simulink model "HILS_ralative"  (R2020a)
settings: Solver=ode4  StartTime=0.0  StopTime=Inf  FixedStep=0.002  RelTol=1e-3
PostLoadFcn:
  | , if any(exist('dsrtsu_mdlpostloadfcn', 'file') == [2, 3, 6]), try dsrtsu_mdlpostloadfcn('Execute', bdroot); catch fprintf('Error in PostLoadFcn (dsrtsu_mdlpostloadfcn) for model "%s":\n %s\n', bdroot, lasterr); end, end,
InitFcn:
  | % mode
  | start_mode = 1;
  | input_mode = 1;
  | HILS_mode = 1;
  | 
  | % input parameter
  | A = 1;
  | Hz = 1;
  | qc = 26500;
  | 
  | % model parameter
  | m1 = 1.5;
  | m2 = 6.4;
  | k1 = 2200;
  | k2 = 405;
  | c1 = 150;
  | c2 = 7;
  | 
  | % convert parameter
  | Gear = 113;
  | enc_pulse = 500;
  | load_to_N = 2;
  | laser_to_mm = 28
  | 
  | % lowpass
  | Cutoff_diff = 20;
  | T_diff = 1/(2*pi*Cutoff_diff);
  | Cutoff_loadcell = 20;
  | T_loadcell = 1/(2*pi*Cutoff_loadcell);
  | Cutoff_laser = 20;
  | T_laser = 1/(2*pi*Cutoff_loadcell);
libraries: rtilib1104 x3, rti1104serlib x2
Description:
  | Standard RTI1104 template.
  | Supported MATLAB version:  R2018a.
settings Model: Tag=RTI1104  DSRTSU_INTERNAL_RTI_VER=520  DSRTSU_INTERNAL_RTI_TYPE=rti1104  RTICANMMDATA=struct('GeneralSetupData',struct('modelroot','C:\Users\VEYRON\Desktop\HILS2020\1DOF_nakagawa\relative','generalsettings',struct('filesettings',struct('destfolder',struct('Name','RTICANMM_FILES','Check',1),'buildfolder',struct('Name','.','Check',1),'AbsDestfolder',struct('Name','C:\Users\VEYRON\Desktop\HILS2020\1DOF_nakagawa\relative\RTICANMM_FILES'),'AbsBuildfolder',struct('Name','C:\Users\VEYRON\Desktop\HILS2020\1DOF_nakagawa\relative'))),'options',struct('addpaths',1,'rmpaths',1,'addtrcexclusion',logical(1),'cannavigator',struct('checkmonitoring',0),'show_usrtrc',0,'use_usrtrc',0),'advanced',struct('options',[1 1 1 1 1 1 1 1 1 1 1 1 1 1 1 1 1 1 1 1 1 1 1 1 1 1 1 1 1 1 1 1 1 1 1 1 1 1 1 1 1 1 1 1 1 1 1 1 1 1 1 1 1 1 1 1 1 1 1 1 1 1 1 1 1 1 1 1 1 1 1 1 1 1 1 1 1 1 1 1 1 1 1 1 1 1 1 1 1 1 1 1 1 1 1 1 1 1 1 1]),'MPSetup',{{}},'modelname','HILS_ralative','block','HILS_ralative'))  DSRTSU_INTERNAL_RTIFLEXRAYCONFIG=110  DSRTSU_INTERNAL_RTIFPGA=110  Creator=VDLAB  LastModifiedBy=Natsu Nakagawa
settings DataIOCC: ReturnWorkspaceOutputs=off
settings OptimizationCC: BlockReduction=off  OptimizeBlockIOStorage=off  BufferReuse=off  GlobalBufferReuse=off  ExpressionFolding=off  LocalBlockOutputs=off  OptimizeDataStoreBuffers=off  BusAssignmentInplaceUpdate=off
settings DebuggingCC: ArithmeticOperatorsInVariantConditions=warning
settings HardwareCC: ProdBitPerPointer=32  ProdBitPerSizeT=32  ProdBitPerPtrDiffT=32  ProdLargestAtomicInteger=Integer  ProdEndianess=BigEndian  ProdWordSize=32  ProdHWDeviceType=Custom Processor->Custom  TargetIntDivRoundTo=Zero  TargetEndianess=BigEndian  TargetHWDeviceType=Custom Processor->Custom
settings SFSimCC: SimUseLocalCustomCode=off  MATLABDynamicMemAlloc=off  CustomCodeUndefinedFunction=UseInterfaceOnly
settings RTWCC: Description=dSPACE DS1104 Hardware Platform  SystemTargetFile=rti1104.tlc  MakeCommand=make_rti  TemplateMakefile=rti1104.tmf  RTWUseLocalCustomCode=off
settings CodeAppCC: StateflowObjectComments=on
settings STFCustomTargetCC: ParMdlRefBuildCompliant=on  SystemTargetFile=rti1104.tlc
settings GRTTargetCC: TargetLangStandard=C89/C90 (ANSI)  CompOptLevelCompliant=off  ConcurrentExecutionCompliant=off  CombineOutputUpdateFcns=off  MatFileLogging=off  CPPClassGenCompliant=off  UseToolchainInfoCompliant=off
settings ConfigComp: CovMetricSettings=dswe

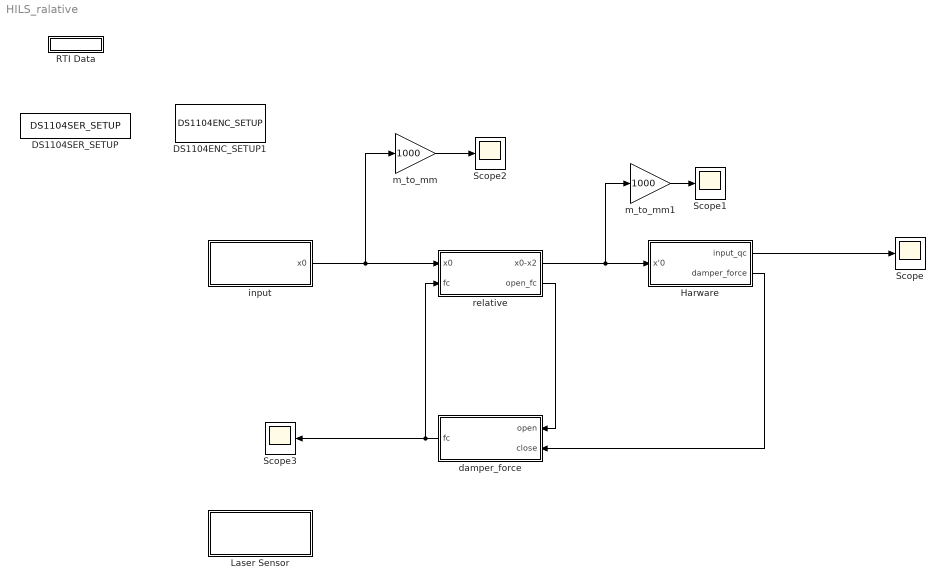
== system HILS_ralative ==
  DS1104ENC_SETUP1 : rtilib1104/DS1104 MASTER PPC/DS1104ENC_SETUP  Reserved1=[]  Reserved2=[]  Reserved3=[]  Reserved4=[]  DialogFcn=gui1104enc_setup  UnitName={'DS1104ENC_SETUP'}  UnitValues={ [] }  DSProperties=struct('RTI',struct('Version',uint32(1),'BlockType',struct('isSLSource',uint8(0),'isSLSink',uint8(0),'isHWSource',uint8(0),'isHWSink',uint8(0),'isSetup',uint8(0),'isInline',uint8(1),'isNonInline',uint8(0),'isInterrupt',uint8(0),'isChannelwise',uint8(0)),'IOBoardType','DS1104MASTER','UnitType','ENC','Identifier','ENCSETUP','DialogType','ML','BlockSet','NONE','SlaveProcessor','NONE'))
      settings: SourceProductName=dSPACE RTI1104  SignalType=[1 1]
  DS1104SER_SETUP : rti1104serlib/DS1104SER_SETUP  Reserved1=[]  Reserved2=[]  Reserved3=[]  Reserved4=[]  DSProperties=struct('RTI',struct('IOBoardType',{{'DS1104','SER'}},'SlaveProcessor','NONE','Version',uint32(2),'BlockType',struct('isSLSource',uint8(0),'isSLSink',uint8(0),'isHWSource',uint8(0),'isHWSink',uint8(0),'isSetup',uint8(1),'isInline',uint8(1),'isNonInline',uint8(0),'isInterrupt',uint8(0),'isChannelwise',uint8(1)),'UnitType','GENSER','Identifier','SETUP','DialogType','ML','BlockSet','NONE'))  RTIBlockInterface=struct('BlockName',struct('Token',{{'DS1104SER_SETUP'}}),'BlockDisplay',{{['Serial Setup'],'center'}},'IconTransparency','off','ParameterTunableNames',{{}},'InitLevel',1,'DialogFcn','guigensersetup','MaskDescription',['To set the global specifications for the UART interface.'])  RTIBlockParameters=struct('ParityMode',{{1,'OFF',[1 5]}},'TransceiverMode',{{1,'OFF',[]}},'QuartzFrequency',{{'16000000','OFF',[1 1]}},'BoardNo',{{1,'ON',[1 1]}},'ChannelNo',{{1,'ON',[1 1]}},'ChannelNumOf',{{1,'OFF',[]}},'BaudRate',{{'115200','OFF',[]}},'DataBitsNumOf',{{4,'OFF',[1 4]}},'StopBitsNumOf',{{1,'OFF',[1 3]}},'ReceiveIntLevelUart',{{4,'OFF',[1 4]}},'AutoflowMode',{{0,'OFF',[]}},'FifoSize',{{'64','OFF',[]}},'ReceiveIntLevelFifo',{{0,'OFF',[]}},'FifoOverrunMode',{{1,'OFF',[]}},'FifoBlockSize',{{'0','OFF',[]}},'TermMode',{{0,'OFF',[]}},'TLCFileName',{{'rtigensersetup','OFF',[]}})  RTISFcnParameters=struct('BoardNo','double','ChannelNo','double','ChannelNumOf','double','BaudRate','double','DataBitsNumOf','double','StopBitsNumOf','double','ParityMode','double','TransceiverMode','double','ReceiveIntLevelUart','double','AutoflowMode','double','FifoSize','double','ReceiveIntLevelFifo','double','FifoBlockSize','double','TermMode','double','QuartzFrequency','double','TLCFileName','char')  RTIBlockParaDefault=struct('ParityMode',1,'TransceiverMode',1,'QuartzFrequency',16000000,'BoardNo',1,'ChannelNo',1,'ChannelNumOf',1,'BaudRate',115200,'DataBitsNumOf',4,'StopBitsNumOf',1,'ReceiveIntLevelUart',4,'AutoflowMode',0,'FifoSize',64,'ReceiveIntLevelFifo',0,'FifoOverrunMode',1,'FifoBlockSize',0,'TermMode',1,'TLCFileName','rtigensersetup')
  Harware : Subsystem
  "Laser Sensor " : Subsystem
  RTI Data : Subsystem  Tag=struct('RTIDataServer',struct('RTIDataServerVs','2','RTIModelDescription','struct(''main'',''HILS_ralative'',''sub'','''',''isMp'',0)'))  LoadFcn="if exist('rtidc'), try,  rtidc('DataHostBlockClbLoad', gcbh); catch, disp(['Warning: ''LoadFcn'' for RTI Data block failed: ' lasterr]); end, end,"  mask(RTI_DATA_HOST){}
      mask help:
      | RTI Data Block.
      | This block is used by RTI to store internal model-dependent data.
      | Please keep this block on the root level of the model. Deleting this block will result in data loss.
      |
      | NEVER DELETE OR COPY THIS BLOCK!
      settings: CopyFcn="if exist('rtidc'), try,  rtidc('DataHostBlockClbCopy', gcbh); catch, disp(['Warning: ''CopyFcn'' for RTI Data block failed: ' lasterr]); end, end,"  DeleteFcn="if exist('rtidc'), try,  rtidc('DataHostBlockClbDelete', gcbh); catch, disp(['Warning: ''DeleteFcn'' for RTI Data block failed: ' lasterr]); end, end,"  ModelCloseFcn="if exist('rtidc'), try,  rtidc('DataHostBlockClbModelClose', gcbh); catch, disp(['Warning: ''ModelCloseFcn'' for RTI Data block failed: ' lasterr]); end, end,"  PreSaveFcn="if exist('rtidc'), try,  rtidc('DataHostBlockClbPreSave', gcbh); catch, disp(['Warning: ''PreSaveFcn'' for RTI Data block failed: ' lasterr]); end, end,"  PostSaveFcn="if exist('rtidc'), try,  rtidc('DataHostBlockClbPostSave', gcbh); catch, disp(['Warning: ''PostSaveFcn'' for RTI Data block failed: ' lasterr]); end, end,"  NameChangeFcn="if exist('rtidc'), try,  rtidc('DataHostBlockClbNameChange', gcbh); catch, disp(['Warning: ''NameChangeFcn'' for RTI Data block failed: ' lasterr]); end, end,"
      mask Help:
      | RTI Data Block.
      | This block is used by RTI to store internal model-dependent data.
      | Please keep this block on the root level of the model. Deleting this block will result in data loss.
      | 
      | NEVER DELETE OR COPY THIS BLOCK!
      mask Display:
      | text(0.5, 0.5, 'RTI Data', 'HorizontalAlignment', 'center');
      | plot([1 0]);
  Scope{,1..3} (4 alike) : Scope
  damper_force : Subsystem
  input : Subsystem
  m_to_mm : Gain  Gain=1000
  m_to_mm1 : Gain  Gain=1000
  relative : Subsystem
  wires:
  input/1(x0) -> m_to_mm/1, relative/1(x0)
  relative/2(open_fc) -> damper_force/1(open)
  damper_force/1(fc) -> Scope3/1, relative/2(fc)
  relative/1(x0-x2) -> m_to_mm1/1, Harware/1(x'0)
  Harware/1(input_qc) -> Scope/1
  Harware/2(damper_force) -> damper_force/2(close)
  m_to_mm/1 -> Scope2/1
  m_to_mm1/1 -> Scope1/1

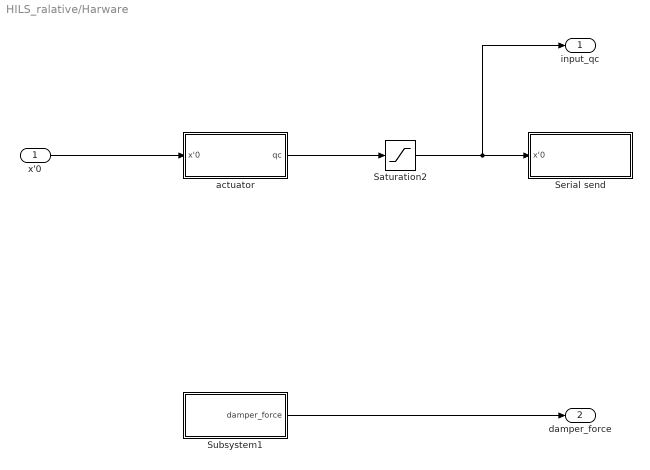
== system HILS_ralative/Harware ==
  x'0 : Inport
  Saturation2 : Saturate  UpperLimit=47000  LowerLimit=0
  Serial send : Subsystem
  Subsystem1 : Subsystem
  actuator : Subsystem
  input_qc : Outport  VectorParamsAs1DForOutWhenUnconnected=off
  damper_force : Outport  Port=2  VectorParamsAs1DForOutWhenUnconnected=off
  wires:
  x'0/1 -> actuator/1(x'0)
  actuator/1(qc) -> Saturation2/1
  Saturation2/1 -> input_qc/1, Serial send/1(x'0)
  Subsystem1/1(damper_force) -> damper_force/1

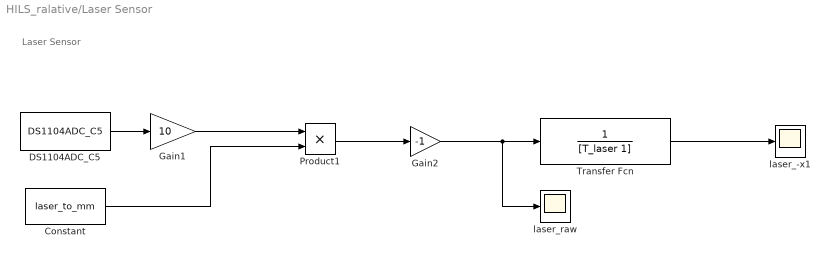
== system HILS_ralative/Laser Sensor  ==
  note: Laser Sensor
  Constant : Constant  Value=laser_to_mm
  DS1104ADC_C5 : rtilib1104/DS1104 MASTER PPC/DS1104ADC_C5  ChannelNo=5  TriggerMode=0  Reserved1=[]  Reserved2=[]  Reserved3=[]  Reserved4=[]  DialogFcn=gui1104adc  UnitName={ 'DS1104ADC_C' }  UnitValues={ 5 }  DSProperties=struct('RTI',struct('Version',uint32(1),'BlockType',struct('isSLSource',uint8(1),'isSLSink',uint8(0),'isHWSource',uint8(1),'isHWSink',uint8(0),'isSetup',uint8(0),'isInline',uint8(1),'isNonInline',uint8(0),'isInterrupt',uint8(0),'isChannelwise',uint8(1)),'IOBoardType','DS1104MASTER','UnitType','ADC','Identifier','ADC','DialogType','ML','BlockSet','NONE','SlaveProcessor','NONE'))
      settings: SourceProductName=dSPACE RTI1104
  Gain1 : Gain  Gain=10
  Gain2 : Gain  Gain=-1
  Product1 : Product
  Transfer Fcn : TransferFcn  Denominator=[T_laser 1]
  laser_-x1 : Scope
  laser_raw : Scope
  wires:
  Gain1/1 -> Product1/1
  Constant/1 -> Product1/2
  DS1104ADC_C5/1 -> Gain1/1
  Product1/1 -> Gain2/1
  Gain2/1 -> laser_raw/1, Transfer Fcn/1
  Transfer Fcn/1 -> laser_-x1/1

== system HILS_ralative/RTI Data ==
  RTI Data Store : Subsystem  Tag="struct('private',struct('version',struct('dsVer',uint32(2),'dsVerCreation',uint32(2),'RTI',struct('ver','7.10','type','RTI1104')),'access',struct('type','Model','isPerm',1,'created',['23-Dec-2020 21:16:23'],'modified',['30-Dec-2020 20:58:09'],'location','')),'public',struct('main',struct('data',[]),'sub',struct('name',{{'HILS_ralative'}},'data',{{struct('TH',struct('thTaskInfo',struct('taskType',{'TIMER','HWINT','TMRINT','SWINT','GLINT'},'tasksNumOf',{1,0,0,0,0},'srcIds',{{'TIMERA'},{},{},{},{}},'taskNames',{{['Timer Task 1']},{},{},{},{}})),'th_tc',struct('dataType','TASK','taskGroupId','','taskGroupList',{{}},'taskSchedulingPolicy','FCFS','taskType','TIMER','blkh',-1,'srcId','TIMERA','srcSgnName',['Timer A interrupt'],'srcCpuName','','taskName',['Timer Task 1  [0.002] s'],'taskNameDisplayExt','','smplTime',0.002,'smplTimeOffs',0,'hasFixedPriority',0,'priority',1,'hasFixedOvc',0,'ovcType',1,'ovcMax',1),'tc_th',struct('dataType','TASK','taskGroupId','','taskGroupList',{{}},'taskSchedulingPolicy','FCFS','taskType','TIMER','blkh',-1,'srcId','TIMERA','srcSgnName',['Timer A interrupt'],'srcCpuName','','taskName',['Timer Task 1  [0.002] s'],'taskNameDisplayExt','','smplTime',0.002,'smplTimeOffs',0,'hasFixedPriority',0,'priority',1,'hasFixedOvc',0,'ovcType',1,'ovcMax',1))}})))"  mask(RTI_DATA_STORE){}
      mask help:
      | RTI Data Store Block. This block is used by RTI to store internal model dependent data. Deleting this block will result in data loss.
      |
      | NEVER DELETE, COPY, OR MODIFY THIS BLOCK!
      mask Help:
      | RTI Data Store Block. This block is used by RTI to store internal model dependent data. Deleting this block will result in data loss.
      | 
      | NEVER DELETE, COPY, OR MODIFY THIS BLOCK!
      mask Display: text(0.5, 0.5, ' ', 'HorizontalAlignment', 'center');

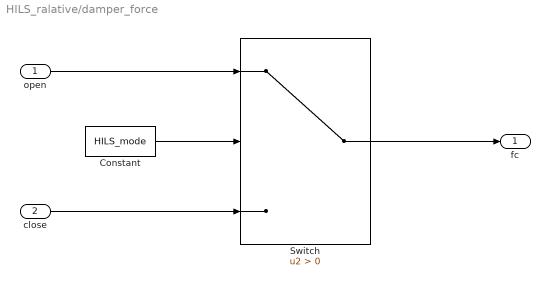
== system HILS_ralative/damper_force ==
  open : Inport
  close : Inport  Port=2
  Constant : Constant  Value=HILS_mode
  Switch : Switch  Criteria=u2 > Threshold
  fc : Outport  VectorParamsAs1DForOutWhenUnconnected=off
  wires:
  open/1 -> Switch/1
  close/1 -> Switch/3
  Constant/1 -> Switch/2
  Switch/1 -> fc/1

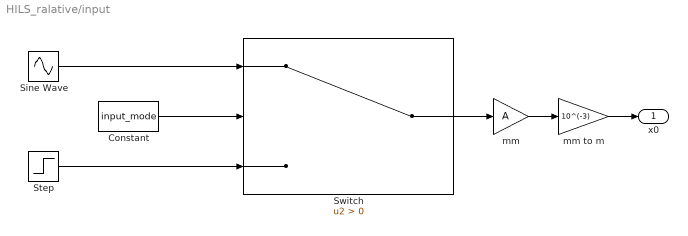
== system HILS_ralative/input ==
  Constant : Constant  Value=input_mode
  Sine Wave : Sin  Frequency=2*pi*Hz  SampleTime=0
  Step : Step  Time=2  SampleTime=0
  Switch : Switch  Criteria=u2 > Threshold
  mm : Gain  Gain=A
  mm to m : Gain  Gain=10^(-3)
  x0 : Outport  VectorParamsAs1DForOutWhenUnconnected=off
  wires:
  Sine Wave/1 -> Switch/1
  Constant/1 -> Switch/2
  Step/1 -> Switch/3
  mm/1 -> mm to m/1
  mm to m/1 -> x0/1
  Switch/1 -> mm/1

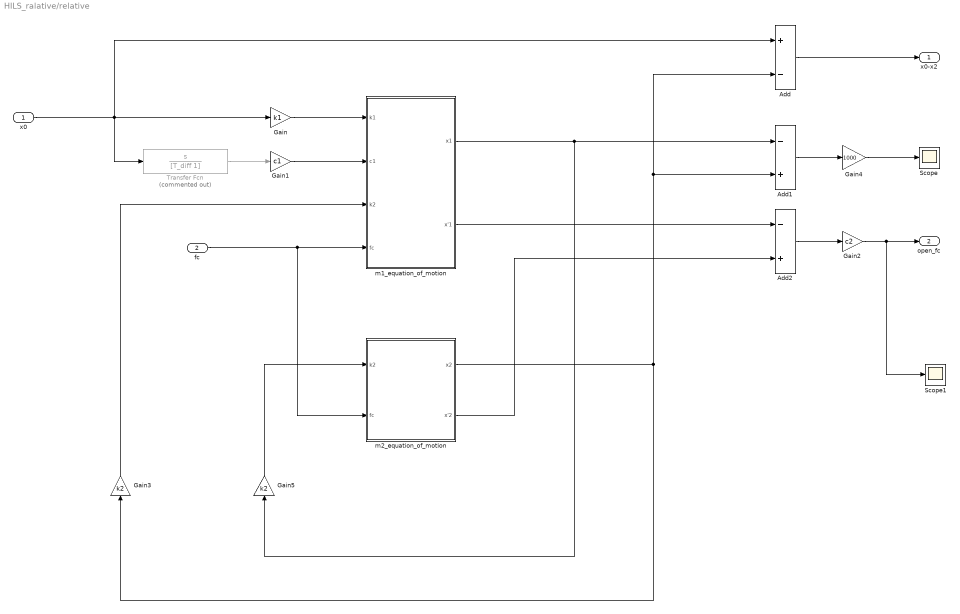
== system HILS_ralative/relative ==
  x0 : Inport
  fc : Inport  Port=2
  Add : Sum  Inputs=+-
  Add1 : Sum  Inputs=-+
  Add2 : Sum  Inputs=-+
  Gain : Gain  Gain=k1
  Gain1 : Gain  Gain=c1
  Gain2 : Gain  Gain=c2
  Gain3 : Gain  Gain=k2
  Gain4 : Gain  Gain=1000
  Gain5 : Gain  Gain=k2
  Scope : Scope
  Scope1 : Scope
  Transfer Fcn : TransferFcn  Commented=on  Numerator=[1 0]  Denominator=[T_diff 1]
  m1_equation_of_motion : Subsystem
  m2_equation_of_motion : Subsystem
  x0-x2 : Outport  VectorParamsAs1DForOutWhenUnconnected=off
  open_fc : Outport  Port=2  VectorParamsAs1DForOutWhenUnconnected=off
  wires:
  x0/1 -> Gain/1, Add/1, Transfer Fcn/1
  Gain/1 -> m1_equation_of_motion/1(k1)
  Transfer Fcn/1 -> Gain1/1
  Gain1/1 -> m1_equation_of_motion/2(c1)
  m2_equation_of_motion/2(x'2) -> Add2/2
  m2_equation_of_motion/1(x2) -> Add1/2, Add/2, Gain3/1
  Gain3/1 -> m1_equation_of_motion/3(k2)
  m1_equation_of_motion/2(x'1) -> Add2/1
  Gain5/1 -> m2_equation_of_motion/1(k2)
  m1_equation_of_motion/1(x1) -> Add1/1, Gain5/1
  Add/1 -> x0-x2/1
  Add1/1 -> Gain4/1
  fc/1 -> m2_equation_of_motion/2(fc), m1_equation_of_motion/4(fc)
  Add2/1 -> Gain2/1
  Gain2/1 -> Scope1/1, open_fc/1
  Gain4/1 -> Scope/1

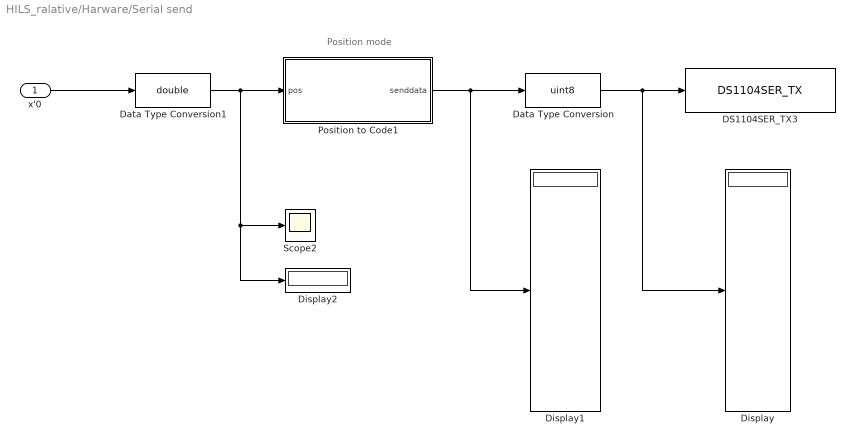
== system HILS_ralative/Harware/Serial send ==
  note: Position mode
  x'0 : Inport
  DS1104SER_TX3 : rti1104serlib/DS1104SER_TX  Reserved1=[]  Reserved2=[]  Reserved3=[]  Reserved4=[]  DSProperties=struct('RTI',struct('IOBoardType',{{'DS1104','SER'}},'SlaveProcessor','NONE','Version',uint32(1),'BlockType',struct('isSLSource',uint8(1),'isSLSink',uint8(1),'isHWSource',uint8(1),'isHWSink',uint8(0),'isSetup',uint8(0),'isInline',uint8(1),'isNonInline',uint8(0),'isInterrupt',uint8(0),'isChannelwise',uint8(1)),'UnitType','GENSER','Identifier','TRANSMIT','DialogType','ML','BlockSet','NONE'))  RTIBlockInterface=struct('BlockName',struct('Token',{{'DS1104SER_TX'}}),'InputPortsWidth',int32([14 1]),'InputPortsActive',[1 0],'InputPortsDataType',{{'SS_UINT8','SS_UINT32'}},'InputPortsName',{{'TXBytes','NumBytes'}},'OutputPortsWidth',int32([1 1]),'OutputPortsActive',[0 0],'OutputPortsDataType',{{'SS_UINT32','SS_INT32'}},'OutputPortsName',{{'NumTXBytes','Status'}},'BlockDisplay',{{['Serial Transmit'],'center'}},'IconTransparency','on','ParameterTunableNames',{{}},'InitLevel',2,'DialogFcn','guigensertransmit','MaskDescription',['To write data to the UART SW FIFO.'])  RTIBlockParameters=struct('BoardNo',{{1,'ON',[1 1]}},'ChannelNo',{{1,'ON',[1 1]}},'ChannelNumOf',{{1,'OFF',[]}},'TransmitFifoOverrunMode',{{1,'OFF',[]}},'ParamTunableMode',{{2,'OFF',[]}},'BytesRefNumOfT',{{'1','OFF',[1 inf]}},'BytesRefNumOfNT',{{'14','OFF',[1 inf]}},'BytesRefNumOfMax',{{'1','OFF',[1 inf]}},'BytesRefNumOfMode',{{0,'OFF',[]}},'BytesActNumOfMode',{{0,'OFF',[]}},'TransmissionStatusMode',{{0,'OFF',[]}},'FifoSizeDefault',{{64,'OFF',[]}},'TLCFileName',{{'rtigensertransmit','OFF',[]}})  RTISFcnParameters=struct('BoardNo','double','ChannelNo','double','ChannelNumOf','double','TransmitFifoOverrunMode','double','ParamTunableMode','double','BytesRefNumOfT','double','BytesRefNumOfNT','double','BytesRefNumOfMax','double','BytesRefNumOfMode','double','BytesActNumOfMode','double','TransmissionStatusMode','double','TLCFileName','char')  RTIBlockParaDefault=struct('BoardNo',1,'ChannelNo',1,'ChannelNumOf',1,'TransmitFifoOverrunMode',1,'ParamTunableMode',1,'BytesRefNumOfT',1,'BytesRefNumOfNT',1,'BytesRefNumOfMax',1,'BytesRefNumOfMode',0,'BytesActNumOfMode',1,'TransmissionStatusMode',1,'FifoSizeDefault',64,'TLCFileName','rtigensertransmit')
  Data Type Conversion : DataTypeConversion  OutDataTypeStr=uint8
  Data Type Conversion1 : DataTypeConversion  OutDataTypeStr=double  RndMeth=Ceiling
  Display : Display
  Display1 : Display
  Display2 : Display
  Position to Code1 : MATLAB Function  TreatAsAtomicUnit=on
  Scope2 : Scope
  wires:
  Data Type Conversion1/1 -> Position to Code1/1(pos), Scope2/1, Display2/1
  Position to Code1/1(senddata) -> Data Type Conversion/1, Display1/1
  Data Type Conversion/1 -> DS1104SER_TX3/1, Display/1
  x'0/1 -> Data Type Conversion1/1

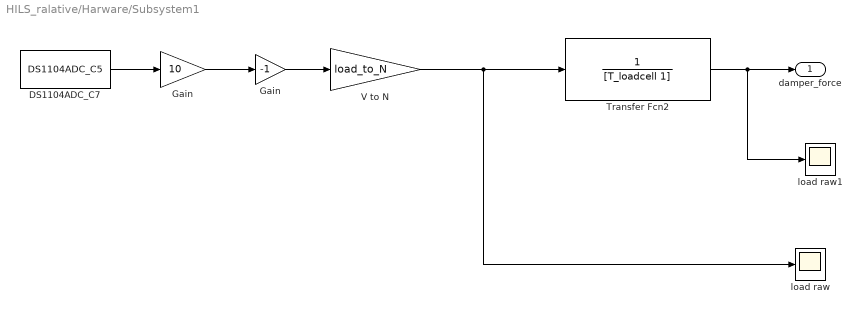
== system HILS_ralative/Harware/Subsystem1 ==
  DS1104ADC_C7 : rtilib1104/DS1104 MASTER PPC/DS1104ADC_C5  ChannelNo=7  TriggerMode=0  Reserved1=[]  Reserved2=[]  Reserved3=[]  Reserved4=[]  DialogFcn=gui1104adc  UnitName={ 'DS1104ADC_C' }  UnitValues={ 7 }  DSProperties=struct('RTI',struct('Version',uint32(1),'BlockType',struct('isSLSource',uint8(1),'isSLSink',uint8(0),'isHWSource',uint8(1),'isHWSink',uint8(0),'isSetup',uint8(0),'isInline',uint8(1),'isNonInline',uint8(0),'isInterrupt',uint8(0),'isChannelwise',uint8(1)),'IOBoardType','DS1104MASTER','UnitType','ADC','Identifier','ADC','DialogType','ML','BlockSet','NONE','SlaveProcessor','NONE'))
      settings: SourceProductName=dSPACE RTI1104
  Gain : Gain  Gain=-1
  "Gain " : Gain  Gain=10
  Transfer Fcn2 : TransferFcn  Denominator=[T_loadcell 1]
  V to N : Gain  Gain=load_to_N
  load raw : Scope
  load raw1 : Scope
  damper_force : Outport  VectorParamsAs1DForOutWhenUnconnected=off
  wires:
  Gain/1 -> V to N/1
  "Gain "/1 -> Gain/1
  DS1104ADC_C7/1 -> "Gain "/1
  V to N/1 -> load raw/1, Transfer Fcn2/1
  Transfer Fcn2/1 -> load raw1/1, damper_force/1

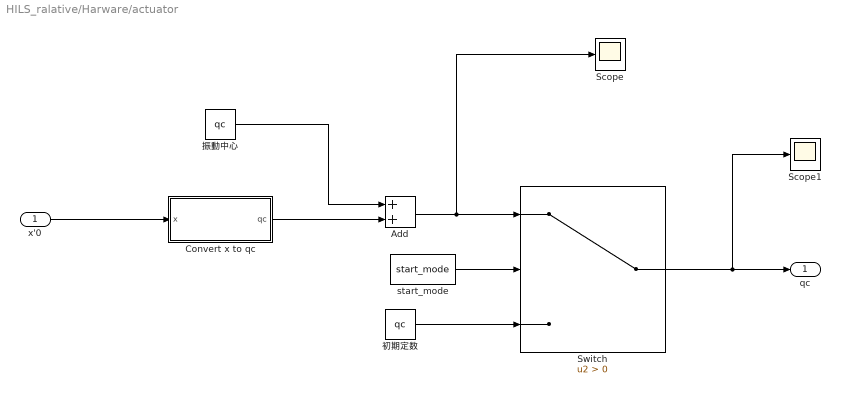
== system HILS_ralative/Harware/actuator ==
  x'0 : Inport
  Add : Sum
  Convert x to qc : Subsystem
  Scope : Scope
  Scope1 : Scope
  Switch : Switch  Criteria=u2 > Threshold
  start_mode : Constant  Value=start_mode
  初期定数 : Constant  Value=qc
  振動中心 : Constant  Value=qc
  qc : Outport  VectorParamsAs1DForOutWhenUnconnected=off
  wires:
  x'0/1 -> Convert x to qc/1(x)
  初期定数/1 -> Switch/3
  Switch/1 -> Scope1/1, qc/1
  start_mode/1 -> Switch/2
  Convert x to qc/1(qc) -> Add/2
  Add/1 -> Scope/1, Switch/1
  振動中心/1 -> Add/1

== system HILS_ralative/RTI Data/RTI Data Store ==
  RTI Data Store : Subsystem  mask(RTI_DATA_STORE){}
      mask help:
      | RTI Data Store Block. This block is used by RTI to store internal model dependent data. Deleting this block will result in data loss.
      |
      | NEVER DELETE, COPY, OR MODIFY THIS BLOCK!
      mask Help:
      | RTI Data Store Block. This block is used by RTI to store internal model dependent data. Deleting this block will result in data loss.
      | 
      | NEVER DELETE, COPY, OR MODIFY THIS BLOCK!
      mask Display: text(0.5, 0.5, ' ', 'HorizontalAlignment', 'center');

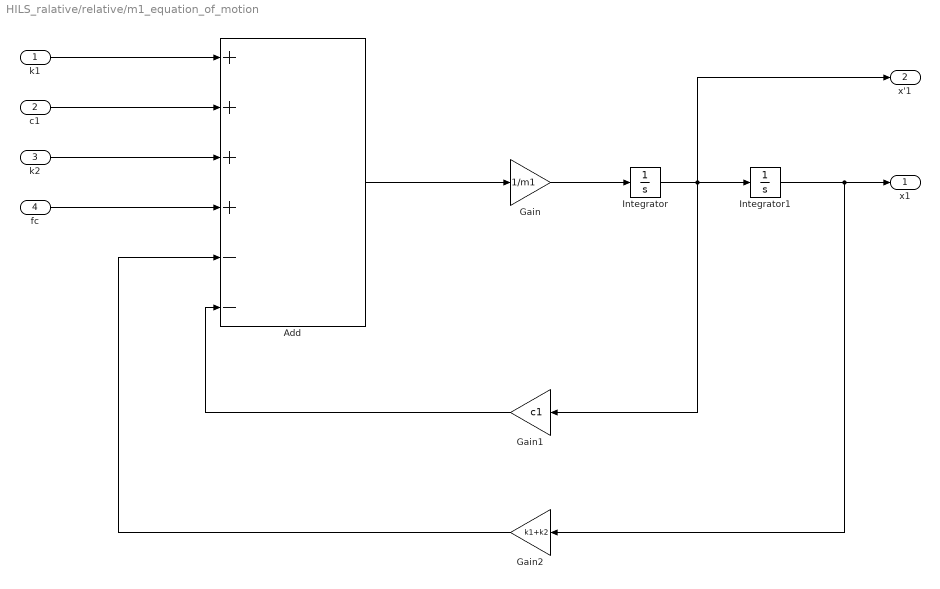
== system HILS_ralative/relative/m1_equation_of_motion ==
  k1 : Inport
  c1 : Inport  Port=2
  k2 : Inport  Port=3
  fc : Inport  Port=4
  Add : Sum  Inputs=++++--
  Gain : Gain  Gain=1/m1
  Gain1 : Gain  Gain=c1
  Gain2 : Gain  Gain=k1+k2
  Integrator : Integrator
  Integrator1 : Integrator
  x1 : Outport  VectorParamsAs1DForOutWhenUnconnected=off
  x'1 : Outport  Port=2  VectorParamsAs1DForOutWhenUnconnected=off
  wires:
  k1/1 -> Add/1
  c1/1 -> Add/2
  k2/1 -> Add/3
  fc/1 -> Add/4
  Add/1 -> Gain/1
  Gain/1 -> Integrator/1
  Integrator/1 -> Integrator1/1, x'1/1, Gain1/1
  Integrator1/1 -> Gain2/1, x1/1
  Gain1/1 -> Add/6
  Gain2/1 -> Add/5

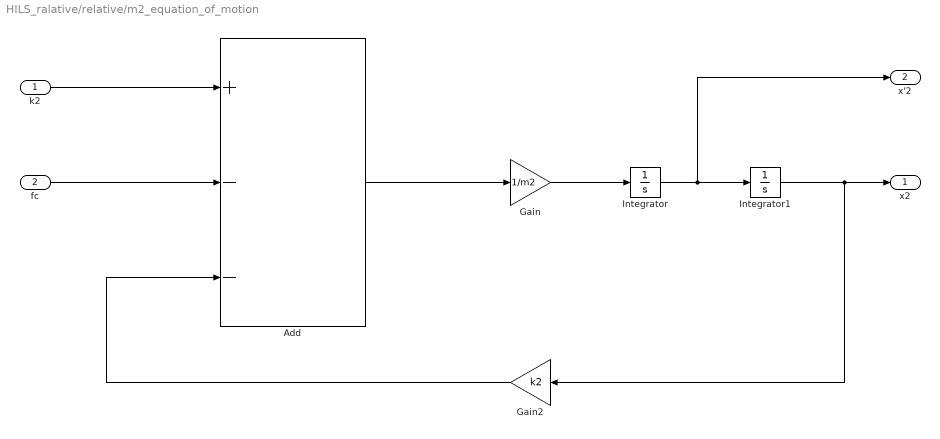
== system HILS_ralative/relative/m2_equation_of_motion ==
  k2 : Inport
  fc : Inport  Port=2
  Add : Sum  Inputs=+--
  Gain : Gain  Gain=1/m2
  Gain2 : Gain  Gain=k2
  Integrator : Integrator
  Integrator1 : Integrator
  x2 : Outport  VectorParamsAs1DForOutWhenUnconnected=off
  x'2 : Outport  Port=2  VectorParamsAs1DForOutWhenUnconnected=off
  wires:
  k2/1 -> Add/1
  fc/1 -> Add/2
  Add/1 -> Gain/1
  Gain/1 -> Integrator/1
  Integrator/1 -> Integrator1/1, x'2/1
  Integrator1/1 -> Gain2/1, x2/1
  Gain2/1 -> Add/3

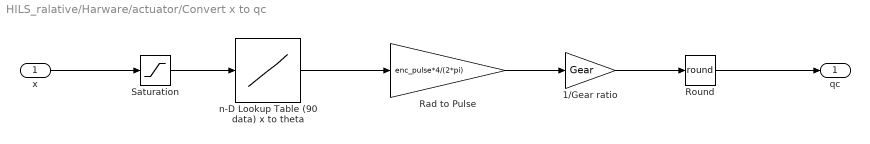
== system HILS_ralative/Harware/actuator/Convert x to qc ==
  x : Inport
  1/Gear ratio : Gain  Gain=Gear
  Rad to Pulse : Gain  Gain=enc_pulse*4/(2*pi)
  Round : Rounding  Operator=round
  Saturation : Saturate  UpperLimit=0.38  LowerLimit=-0.25
  n-D Lookup Table (90 data) x to theta : Lookup_n-D  NumberOfTableDimensions=1  BreakpointsForDimension1=|  BreakpointsForDimension3=[5, 7]  Table=|  InterpMethod=Cubic spline  ExtrapMethod=Cubic spline  InternalRulePriority=Speed  RndMeth=Simplest  InputSameDT=on
      BreakpointsForDimension1=|
      | [-0.0255748
      | -0.025224748
      | -0.024865444
      | -0.024496806
      | -0.024118754
      | -0.023731207
      | -0.023334088
      | -0.022927321
      | -0.022510829
      | -0.022084541
      | -0.021648387
      | -0.021202299
      | -0.020746214
      | -0.02028007
      | -0.01980381
      | -0.019317383
      | -0.018820738
      | -0.018313834
      | -0.01779663
      | -0.017269095
      | -0.016731201
      | -0.016182927
      | -0.015624258
      | -0.015055189
      | -0.014475717
      | -0.013885852
      | -0.013285608
      | -0.012675011
      | -0.012054093
      | -0.011422895
      | -0.010781471
      | -0.01012988
      | -0.009468194
      | -0.008796496
      | -0.008114876
      | -0.007423439
      | -0.006722299
      | -0.006011582
      | -0.005291424
      | -0.004561974
      | -0.003823394
      | -0.003075856
      | -0.002319545
      | -0.001554657
      | -0.000781402
      | 0
      | 0.000789315
      | 0.001586298
      | 0.002390691
      | 0.003202226
      | 0.004020623
      | 0.004845587
      | 0.005676817
      | 0.006513997
      | 0.007356803
      | 0.008204897
      | 0.009057933
      | 0.009915556
      | 0.010777401
      | 0.011643091
      | 0.012512243
      | 0.013384467
      | 0.014259361
      | 0.015136519
      | 0.016015526
      | 0.016895961
      | 0.017777398
      | 0.018659405
      | 0.019541543
      | 0.020423371
      | 0.021304443
      | 0.022184308
      | 0.023062515
      | 0.023938607
      | 0.024812127
      | 0.025682617
      | 0.026549617
      | 0.027412664
      | 0.0282713
      | 0.029125062
      | 0.029973492
      | 0.030816132
      | 0.031652523
      | 0.032482212
      | 0.033304747
      | 0.034119678
      | 0.034926559
      | 0.035724949
      | 0.036514409
      | 0.037294505
      | 0.03806481
      | ]
      Table=|
      | [-0.785398163
      | -0.767944871
      | -0.750491578
      | -0.733038286
      | -0.715584993
      | -0.698131701
      | -0.680678408
      | -0.663225116
      | -0.645771823
      | -0.628318531
      | -0.610865238
      | -0.593411946
      | -0.575958653
      | -0.558505361
      | -0.541052068
      | -0.523598776
      | -0.506145483
      | -0.488692191
      | -0.471238898
      | -0.453785606
      | -0.436332313
      | -0.41887902
      | -0.401425728
      | -0.383972435
      | -0.366519143
      | -0.34906585
      | -0.331612558
      | -0.314159265
      | -0.296705973
      | -0.27925268
      | -0.261799388
      | -0.244346095
      | -0.226892803
      | -0.20943951
      | -0.191986218
      | -0.174532925
      | -0.157079633
      | -0.13962634
      | -0.122173048
      | -0.104719755
      | -0.087266463
      | -0.06981317
      | -0.052359878
      | -0.034906585
      | -0.017453293
      | 0
      | 0.017453293
      | 0.034906585
      | 0.052359878
      | 0.06981317
      | 0.087266463
      | 0.104719755
      | 0.122173048
      | 0.13962634
      | 0.157079633
      | 0.174532925
      | 0.191986218
      | 0.20943951
      | 0.226892803
      | 0.244346095
      | 0.261799388
      | 0.27925268
      | 0.296705973
      | 0.314159265
      | 0.331612558
      | 0.34906585
      | 0.366519143
      | 0.383972435
      | 0.401425728
      | 0.41887902
      | 0.436332313
      | 0.453785606
      | 0.471238898
      | 0.488692191
      | 0.506145483
      | 0.523598776
      | 0.541052068
      | 0.558505361
      | 0.575958653
      | 0.593411946
      | 0.610865238
      | 0.628318531
      | 0.645771823
      | 0.663225116
      | 0.680678408
      | 0.698131701
      | 0.715584993
      | 0.733038286
      | 0.750491578
      | 0.767944871
      | 0.785398163
      | ]
  qc : Outport  VectorParamsAs1DForOutWhenUnconnected=off
  wires:
  x/1 -> Saturation/1
  Saturation/1 -> n-D Lookup Table (90 data) x to theta/1
  n-D Lookup Table (90 data) x to theta/1 -> Rad to Pulse/1
  Rad to Pulse/1 -> 1/Gear ratio/1
  1/Gear ratio/1 -> Round/1
  Round/1 -> qc/1

== system HILS_ralative/RTI Data/RTI Data Store/RTI Data Store ==
  RTI Data Store : Subsystem  mask(RTI_DATA_STORE){}
      mask help:
      | RTI Data Store Block. This block is used by RTI to store internal model dependent data. Deleting this block will result in data loss.
      |
      | NEVER DELETE, COPY, OR MODIFY THIS BLOCK!
      mask Help:
      | RTI Data Store Block. This block is used by RTI to store internal model dependent data. Deleting this block will result in data loss.
      | 
      | NEVER DELETE, COPY, OR MODIFY THIS BLOCK!
      mask Display: text(0.5, 0.5, ' ', 'HorizontalAlignment', 'center');

== system HILS_ralative/RTI Data/RTI Data Store/RTI Data Store/RTI Data Store ==
  RTI Data Store : Subsystem  mask(RTI_DATA_STORE){}
      mask help:
      | RTI Data Store Block. This block is used by RTI to store internal model dependent data. Deleting this block will result in data loss.
      |
      | NEVER DELETE, COPY, OR MODIFY THIS BLOCK!
      mask Help:
      | RTI Data Store Block. This block is used by RTI to store internal model dependent data. Deleting this block will result in data loss.
      | 
      | NEVER DELETE, COPY, OR MODIFY THIS BLOCK!
      mask Display: text(0.5, 0.5, ' ', 'HorizontalAlignment', 'center');

== system HILS_ralative/RTI Data/RTI Data Store/RTI Data Store/RTI Data Store/RTI Data Store ==

== matlab function HILS_ralative/Harware/Serial send/Position to Code1 ==
  data: pos input; senddata output
% script_sendTargetPosition
% MATLAB EPOS LibraryのsendTargetPosition()から書き換え

% function [] = sendTargetPosition( obj, pos )

function senddata = func_sendTargetPosition(pos)
% pos = 20480;

%Sets the TargetPosition for Profile Position mode
%pos must be an integer.
pos_hex = '';

if pos >= 0
    pos_hex = dec2hex(pos, 8);
else
    pos_hex = dec2hex(2^32+pos, 8);
end

%% Build write object request frame EPOS Node 1
%opCode(write): 0x11
%Len-1: 3
%object index(Target Position): 0x2062
%subindex and nodeID: 0x0100
%BYTE Data[4]: pos_hex(1:4), pos_hex(5:8)


%opCode = uint16(myhex2dec('11'));
opCode = uint16(17);
Len_1 = uint16(3);
%DATA = uint16([myhex2dec('62') myhex2dec('20') myhex2dec('00') myhex2dec('01') myhex2dec(pos_hex(7:8))
%   myhex2dec(pos_hex(5:6)) 
%   myhex2dec(pos_hex(3:4)) myhex2dec(pos_hex(1:2)) ]);
DATA = uint16([98 32 0 1 myhex2dec(pos_hex(7:8)) myhex2dec(pos_hex(5:6)) myhex2dec(pos_hex(3:4)) myhex2dec(pos_hex(1:2)) ]);
%DATAforCRC = uint16([myhex2dec('1103') myhex2dec('2062') myhex2dec('0100') myhex2dec(pos_hex(5:8)) 
%   myhex2dec(pos_hex(1:4)) myhex2dec('0000')]);
DATAforCRC = uint16([4355 8290 256 myhex2dec(pos_hex(5:8)) myhex2dec(pos_hex(1:4)) 0]);
numberofWordsCRC = 6;
crc_hex = dec2hex(CRCcalc(DATAforCRC, numberofWordsCRC),4);
CRC = uint16([myhex2dec(crc_hex(3:4)) myhex2dec(crc_hex(1:2))]);

% senddata=[opCode Len_1 DATA CRC char('O')];
senddata=[opCode Len_1 DATA CRC 79 10]';

end


function d = myhex2dec(h)
%HEX2DEC Convert hexadecimal string to decimal integer.
%   this is the hex2dec function from Matlab with some checking disabled
%   for faster performance

if iscellstr(h), h = char(h); end
if isempty(h), d = []; return, end

% Work in upper case. - disabled since upper case anyways
%h = upper(h);

[m,n]=size(h);

% Right justify strings and form 2-D character array.
if ~isempty(find((h==' ' | h==0),1))
  h = strjust(h);

  % Replace any leading blanks and nulls by 0.
  h(cumsum(h ~= ' ' & h ~= 0,2) == 0) = '0';
else
  h = reshape(h,m,n);
end

% Check for out of range values - disabled
% if any(any(~((h>='0' & h<='9') | (h>='A'&h<='F'))))
%    error(message('MATLAB:hex2dec:IllegalHexadecimal'));
% end

sixteen = 16;
p = fliplr(cumprod([1 sixteen(ones(1,n-1))]));
p = p(ones(m,1),:);

d = h <= 64; % Numbers
h(d) = h(d) - 48;

d =  h > 64; % Letters
h(d) = h(d) - 55;

d = sum(h.*p,2);


end

function [ CRC ] = CRCcalc(DataArray, CRCnumberOfWords)
%Calculates the 16 bit CRC checksum according to communication guide for
%EPOS2
%Arguments are the DataArray that is being sent (opCode to Data) and the
%number of words

CRC = uint16(0);
for i=1:CRCnumberOfWords
    
    %shifter = uint16(myhex2dec('8000'));
    shifter = uint16(32768);
    c = DataArray(i);
    
    while(shifter)
        %carry = bitand(CRC, uint16(myhex2dec('8000')), 'uint16');
        carry = bitand(CRC, uint16(32768), 'uint16');
        CRC = bitshift(CRC,1,'uint16');
        if(bitand(c, shifter, 'uint16'))
            CRC = CRC +  1;
        end
        if(carry)
            %CRC = bitxor(CRC,uint16(myhex2dec('1021')),'uint16');
            CRC = bitxor(CRC,uint16(4129),'uint16');
        end
        shifter = bitshift(shifter,-1,'uint16');
    end
    
end


end
